simulink model "GIL11_slow_mechanism"  (R2023b)
settings: Solver=FixedStepAuto  StartTime=0.233  StopTime=1.3573  FixedStep=0.01  RelTol=1e-3
PreLoadFcn:
  | kinData_max = 0;
  | kinData_min = 0;
libraries: simulink x2
settings Model: Creator=admin-local  LastModifiedBy=admin-local
settings SolverCC: AlgebraicLoopSolver=TrustRegion
settings DebuggingCC: UnconnectedInputMsg=warning  UnconnectedOutputMsg=warning  UnconnectedLineMsg=warning
settings ModelReferenceCC: EnableRefExpFcnMdlSchedulingChecks=on

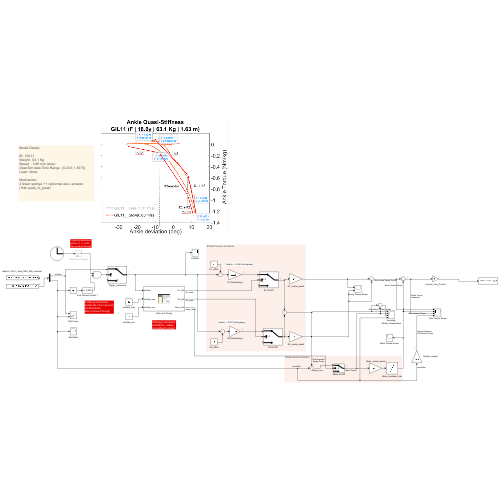
[thumbnail: Simulink's stored preview of the top-level diagram]
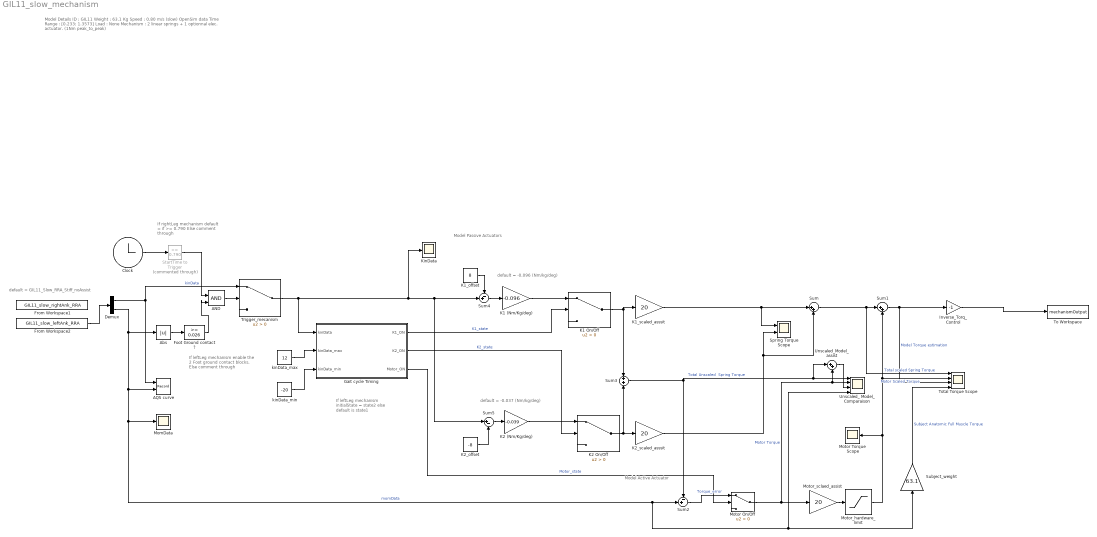
== system GIL11_slow_mechanism ==
  note: Model Passive Actuators
  note: default = -0.096 (Nm/kg/deg)
  note: default = -0.037 (Nm/kg/deg)
  note: Model Active Actuator
  note: default = GIL11_Slow_RRA_Stiff_noAssist
  note: Model Details
      |
      | ID : GIL11
      | Weight : 63.1 Kg
      | Speed  : 0.80 m/s (slow)
      | OpenSim data Time Range : [0.233; 1.3573]
      | Load : None
      |
      | Mechanism :
      | 2 linear springs + 1 optionnal elec. actuator.
      | (1Nm peak_to_peak)
  note: If leftLeg mechanism
      | enable the 2 Foot ground contact blocks.
      | Else comment through
  note: If rightLeg mechanism
      | default = if  >= 0.790
      | Else comment through
  note: If leftLeg mechanism
      | initialState = state2
      | else default is state1
  AND : Logic  IconShape=distinctive  AllPortsSameDT=off  OutDataTypeStr=boolean
  AQS curve : Record  FileSettingsInternal="{\"entries\":[{\"content\":{\"excelSettings\":{\"content\":{},\"type\":\"Streamout.ExcelSettings\"}},\"type\":\"Streamout.FileSettingStorage\",\"uuid\":\"\"}],\"packageUris\":[\"http:\\/\\/schema.mathworks.com\\/mf0\\/streamout_blocks\\/R2020a\"],\"version\":\"1.0\"}"  Layout=[1 1]  SignalsInternal="{\"entries\":[{\"content\":{\"signals\":[{\"content\":{\"blockPath\":[],\"dimensions\":[1],\"domain\":\"\",\"lineColor\":\"#64d413\",\"port\":1,\"sid\":[\"\"],\"signalID\":1,\"signalName\":\"kinData\"},\"type\":\"RecordBlkView.Signal\",\"uuid\":\"\"},{\"content\":{\"blockPath\":[],\"dimensions\":[1],\"domain\":\"\",\"lineColor\":\"#ff13a6\",\"port\":2,\"sid\":[\"\"],\"signalID\":2,\"signalName\":\"momData\"},\"type\":\"RecordBlkView.Signal\",\"uuid\":\"\"}]},\"type\":\"RecordBlkView.InputSignals\",\"uuid\":\"\"}],\"packageUris\":[\"http:\\/\\/schema.mathworks.com\\/mf0\\/streamout_blocks\\/R2020a\"],\"version\":\"1.0\"}"  VisualizationBindings="{\"xyplotplugin\":{\"info\":[{\"series\":[],\"subplotID\":1}]}}"  CompatibilityTag=XY  st=-1
  Abs : Abs  SaturateOnIntegerOverflow=off
  Clock : Clock
  Demux : Demux  Outputs=2
  Foot Ground contact ? : simulink/Logic and Bit Operations/Compare To Constant  relop=>=  const=0.026  OutDataTypeStr=boolean
  From Workspace1 : FromWorkspace  VariableName=GIL11_slow_rightAnk_RRA  OutputAfterFinalValue=Holding final value
  From Workspace2 : FromWorkspace  VariableName=GIL11_slow_leftAnk_RRA  OutputAfterFinalValue=Holding final value
  Gait cycle Timing : State Transition Table  TreatAsAtomicUnit=on
  Inverse_Torq_Control : Gain  Gain=-1
  K1 (Nm/Kg/deg) : Gain  Gain=-0.096
  K1 On/Off : Switch  Criteria=u2 > Threshold  SaturateOnIntegerOverflow=off  InputSameDT=off
  "K1_offset " : Constant  Value=8
  K1_scaled_asssit : Gain  Gain=20
  K2 (Nm/Kg/deg) : Gain  Gain=-0.039
  K2 On/Off : Switch  Criteria=u2 > Threshold  SaturateOnIntegerOverflow=off  InputSameDT=off
  K2_offset : Constant  Value=-8
  K2_scaled_asssit : Gain  Gain=20
  KinData : Scope
  "MomData " : Scope
  Motor On/Off : Switch  Criteria=u2 > Threshold  SaturateOnIntegerOverflow=off  InputSameDT=off
  Motor Torque Scope : Scope
  Motor_hardware_limit : Saturate  UpperLimit=16  LowerLimit=-16
  Motor_sclaed_assist : Gain  Gain=20
  Spring Torque Scope : Scope  NumInputPorts=2
  StartTime to Trigger : simulink/Logic and Bit Operations/Compare To Constant  Commented=through  relop=>=  const=0.790  OutDataTypeStr=boolean
  Subject_weight : Gain  Gain=63.1
  Sum : Sum  Inputs=|++
  Sum1 : Sum  Inputs=|++
  Sum2 : Sum  Inputs=-+|
  Sum3 : Sum  Inputs=+|+
  Sum4 : Sum  Inputs=-+|
  Sum5 : Sum  Inputs=|+-
  To Workspace : ToWorkspace  VariableName=mechanismOutput  SaveFormat=Timeseries  SampleTime=-1
  Total Torque Scope : Scope  NumInputPorts=4
  Trigger_mecanism : Switch  Criteria=u2 > Threshold  SaturateOnIntegerOverflow=off  InputSameDT=off
  Unscaled_ Model_Comparaison : Scope  NumInputPorts=4
  Unscaled_Model_assist : Sum  Inputs=|++
  "kinData_max " : Constant  Value=12
  "kinData_min " : Constant  Value=-20
  wires:
  Gait cycle Timing/1(K1_ON) -> K1 On/Off/2  "K1_state"
  Motor On/Off/1 -> Unscaled_Model_assist/2, Unscaled_ Model_Comparaison/2, Motor_sclaed_assist/1  "Motor Torque"
  Gait cycle Timing/2(K2_ON) -> K2 On/Off/2  "K2_state"
  "kinData_max "/1 -> Gait cycle Timing/2(kinData_max)
  Gait cycle Timing/3(Motor_ON) -> Motor On/Off/2  "Motor_state"
  Demux/1 -> Trigger_mecanism/1, AQS curve/1  "kinData"
  Sum2/1 -> Motor On/Off/1  "Torque_error"
  Sum1/1 -> Total Torque Scope/3, Inverse_Torq_Control/1  "Model Torque estimation"
  K1_scaled_asssit/1 -> Spring Torque Scope/1, Sum/1
  "kinData_min "/1 -> Gait cycle Timing/3(kinData_min)
  Demux/2 -> AQS curve/2, "MomData "/1, Subject_weight/1, Unscaled_ Model_Comparaison/4, Sum2/2, Abs/1  "momData"
  "K1_offset "/1 -> Sum4/1
  K2_offset/1 -> Sum5/2
  K1 On/Off/1 -> K1_scaled_asssit/1, Sum3/1
  Sum4/1 -> K1 (Nm/Kg/deg)/1
  Sum5/1 -> K2 (Nm/Kg/deg)/1
  K2 On/Off/1 -> K2_scaled_asssit/1, Sum3/2
  K1 (Nm/Kg/deg)/1 -> K1 On/Off/1
  K2 (Nm/Kg/deg)/1 -> K2 On/Off/1
  Subject_weight/1 -> Total Torque Scope/4  "Subject Anatomic Full Muscle Torque"
  Sum3/1 -> Unscaled_Model_assist/1, Unscaled_ Model_Comparaison/1, Sum2/1  "Total Unscaled  Spring Torque"
  K2_scaled_asssit/1 -> Spring Torque Scope/2, Sum/2
  Sum/1 -> Total Torque Scope/1, Sum1/1  "Total scaled Spring Torque"
  Motor_hardware_limit/1 -> Total Torque Scope/2, Sum1/2, Motor Torque Scope/1  "Motor Scaled Torque"
  Motor_sclaed_assist/1 -> Motor_hardware_limit/1
  Trigger_mecanism/1 -> KinData/1, Sum4/2, Sum5/1, Gait cycle Timing/1(kinData)
  Unscaled_Model_assist/1 -> Unscaled_ Model_Comparaison/3
  Clock/1 -> StartTime to Trigger/1
  StartTime to Trigger/1 -> AND/1
  Foot Ground contact ?/1 -> AND/2
  AND/1 -> Trigger_mecanism/2
  Abs/1 -> Foot Ground contact ?/1
  Inverse_Torq_Control/1 -> To Workspace/1
  From Workspace2/1 -> Demux/1

== stateflow chart GIL11_slow_mechanism/Gait cycle Timing ==
  state state1
    K2_ON = 0
  state state2
    K2_ON = 1
  state state3
  state state4
  state state5
  state state6
  (junction 284) -> state1
  (junction 286) -> (junction 284)
  state1 -> state2 : [kinData <= -8 & K2_ON == 0]
      | {K1_ON= 0;
      | K2_ON = 1;
      | Motor_ON = 0;}
  (default) -> state2
  state2 -> (junction 269) [order 2] : [kinData > -6 & kinData <= -5 ]
      | {K1_ON= 0;
      | K2_ON = 0;
      | Motor_ON = 0;}
  (junction 269) -> state2
  state2 -> state3 [order 1] : [kinData > 8]
      | {K1_ON= 1;
      | K2_ON = 1;
      | Motor_ON = 0;}
  state3 -> state4 : [kinData >= kinData_max]
      | {K1_ON= 1;
      | K2_ON = 1;
      | Motor_ON = 1;}
  state4 -> state5 : [kinData <= 8]
      | {K1_ON= 0;
      | K2_ON = 1;
      | Motor_ON = 1;}
  state5 -> state6 : [[kinData <= -8]]
      | {K1_ON= 0;
      | K2_ON = 0;
      | Motor_ON = 1;}
  state6 -> (junction 286) : [kinData <= kinData_min]
      | {K1_ON= 0;
      | K2_ON = 0;
      | Motor_ON = 0;}
  data: kinData input; K1_ON output; K2_ON output; Motor_ON output; kinData_max input; kinData_min input
